simulink model "SOC_Battery"  (R2013a)
settings: Solver=ode45  StartTime=0.0  StopTime=10.0  RelTol=1e-3
libraries: simulink x11
settings Model: Creator=Admin  LastModifiedBy=Admin

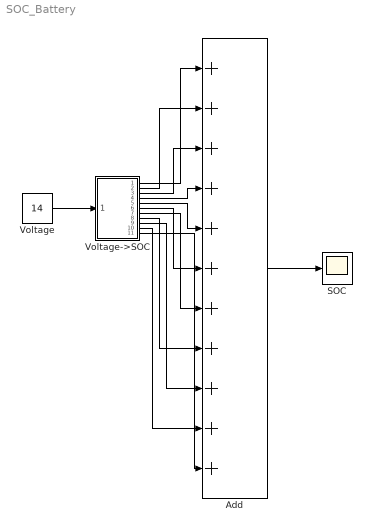
== system SOC_Battery ==
  Add : Sum  Inputs=+++++++++++
  "SOC " : Scope
  Voltage : Constant  Value=14
  Voltage->SOC : Subsystem
  wires:
  Add/1 -> "SOC "/1
  Voltage/1 -> Voltage->SOC/1(In1)
  Voltage->SOC/1(Out1) -> Add/1
  Voltage->SOC/2(Out2) -> Add/2
  Voltage->SOC/3(Out3) -> Add/3
  Voltage->SOC/4(Out4) -> Add/4
  Voltage->SOC/5(Out5) -> Add/5
  Voltage->SOC/6(Out6) -> Add/6
  Voltage->SOC/7(Out7) -> Add/7
  Voltage->SOC/8(Out8) -> Add/8
  Voltage->SOC/9(Out9) -> Add/9
  Voltage->SOC/10(Out10) -> Add/10
  Voltage->SOC/11(Out11) -> Add/11

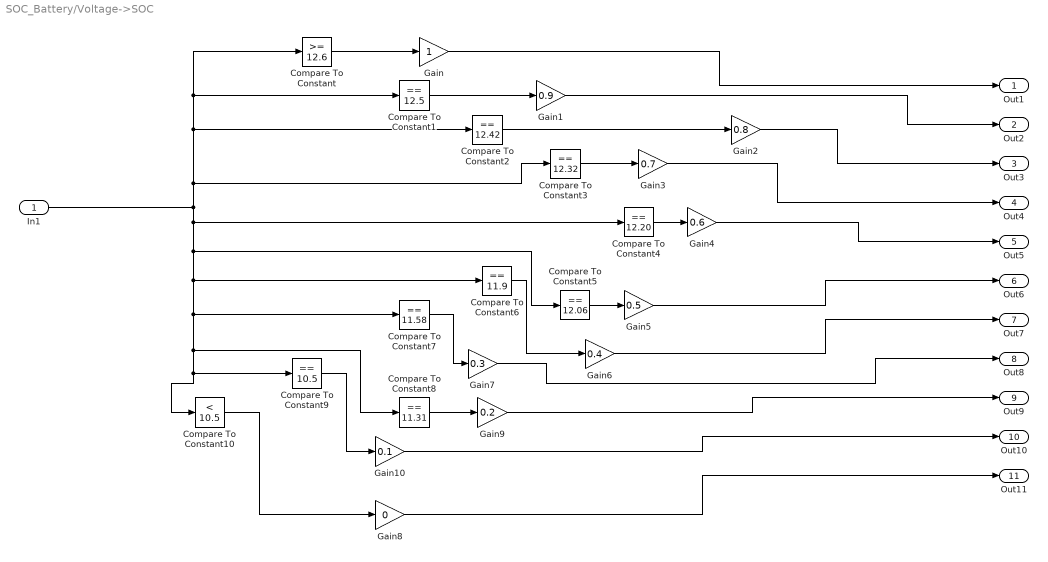
== system SOC_Battery/Voltage->SOC ==
  In1 : Inport
  Compare To Constant : simulink/Logic and Bit Operations/Compare To Constant  relop=>=  const=12.6  OutDataTypeStr=boolean
  Compare To Constant1 : simulink/Logic and Bit Operations/Compare To Constant  relop===  const=12.5  OutDataTypeStr=boolean
  Compare To Constant10 : simulink/Logic and Bit Operations/Compare To Constant  relop=<  const=10.5  OutDataTypeStr=boolean
  Compare To Constant2 : simulink/Logic and Bit Operations/Compare To Constant  relop===  const=12.42  OutDataTypeStr=boolean
  Compare To Constant3 : simulink/Logic and Bit Operations/Compare To Constant  relop===  const=12.32  OutDataTypeStr=boolean
  Compare To Constant4 : simulink/Logic and Bit Operations/Compare To Constant  relop===  const=12.20  OutDataTypeStr=boolean
  Compare To Constant5 : simulink/Logic and Bit Operations/Compare To Constant  relop===  const=12.06  OutDataTypeStr=boolean
  Compare To Constant6 : simulink/Logic and Bit Operations/Compare To Constant  relop===  const=11.9  OutDataTypeStr=boolean
  Compare To Constant7 : simulink/Logic and Bit Operations/Compare To Constant  relop===  const=11.58  OutDataTypeStr=boolean
  Compare To Constant8 : simulink/Logic and Bit Operations/Compare To Constant  relop===  const=11.31  OutDataTypeStr=boolean
  Compare To Constant9 : simulink/Logic and Bit Operations/Compare To Constant  relop===  const=10.5  OutDataTypeStr=boolean
  Gain : Gain
  Gain1 : Gain  Gain=0.9
  Gain10 : Gain  Gain=0.1
  Gain2 : Gain  Gain=0.8
  Gain3 : Gain  Gain=0.7
  Gain4 : Gain  Gain=0.6
  Gain5 : Gain  Gain=0.5
  Gain6 : Gain  Gain=0.4
  Gain7 : Gain  Gain=0.3
  Gain8 : Gain  Gain=0
  Gain9 : Gain  Gain=0.2
  Out1 : Outport
  Out2 : Outport  Port=2
  Out3 : Outport  Port=3
  Out4 : Outport  Port=4
  Out5 : Outport  Port=5
  Out6 : Outport  Port=6
  Out7 : Outport  Port=7
  Out8 : Outport  Port=8
  Out9 : Outport  Port=9
  Out10 : Outport  Port=10
  Out11 : Outport  Port=11
  wires:
  In1/1 -> Compare To Constant6/1, Compare To Constant8/1, Compare To Constant9/1, Compare To Constant10/1, Compare To Constant7/1, Compare To Constant5/1, Compare To Constant4/1, Compare To Constant2/1, Compare To Constant1/1, Compare To Constant/1, Compare To Constant3/1
  Compare To Constant/1 -> Gain/1
  Compare To Constant1/1 -> Gain1/1
  Compare To Constant2/1 -> Gain2/1
  Compare To Constant3/1 -> Gain3/1
  Compare To Constant4/1 -> Gain4/1
  Compare To Constant5/1 -> Gain5/1
  Compare To Constant6/1 -> Gain6/1
  Compare To Constant7/1 -> Gain7/1
  Compare To Constant8/1 -> Gain9/1
  Compare To Constant9/1 -> Gain10/1
  Compare To Constant10/1 -> Gain8/1
  Gain/1 -> Out1/1
  Gain1/1 -> Out2/1
  Gain2/1 -> Out3/1
  Gain3/1 -> Out4/1
  Gain4/1 -> Out5/1
  Gain5/1 -> Out6/1
  Gain6/1 -> Out7/1
  Gain7/1 -> Out8/1
  Gain9/1 -> Out9/1
  Gain10/1 -> Out10/1
  Gain8/1 -> Out11/1
